simulink model "gm_sampleModel1708_2_sub"  (R2023a)
settings: Solver=VariableStepAuto  StartTime=0.0  StopTime=10.0  RelTol=1e-3
libraries: simulink x4, hdlsllib x1
settings Model: Creator=user1  LastModifiedBy=user1
settings OptimizationCC: BlockReduction=off  ConditionallyExecuteInputs=off
settings DebuggingCC: InheritedTsInSrcMsg=none

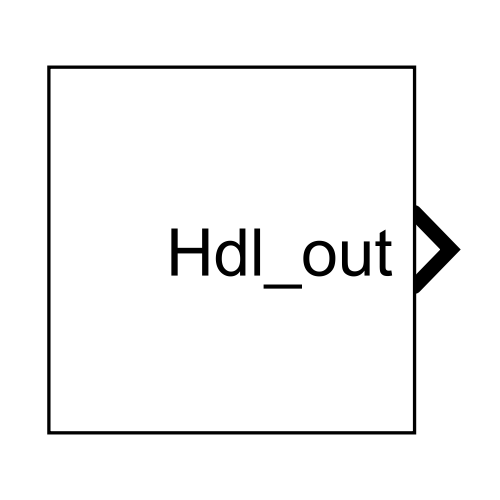
[thumbnail: Simulink's stored preview of the top-level diagram]
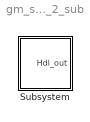
== system gm_sampleModel1708_2_sub ==
  Subsystem : Subsystem

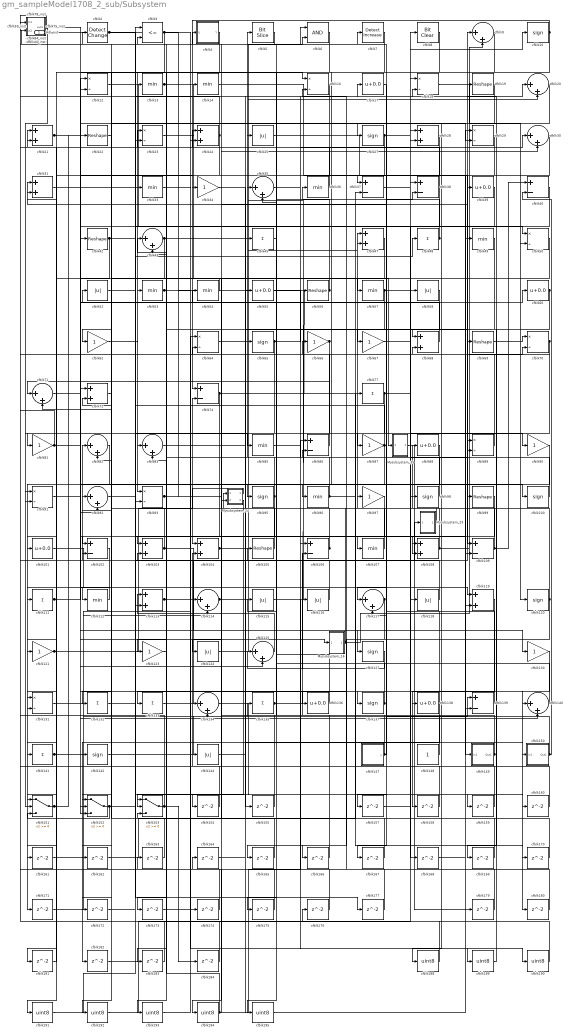
== system gm_sampleModel1708_2_sub/Subsystem ==
  Mysubsystem_16 : Subsystem
  Mysubsystem_23 : Subsystem
  Mysubsystem_24 : Subsystem
  Mysubsystem_35 : Subsystem
  cfblk{10,27,65,95,98,100,120,127,137,142} (10 alike) : Signum
  cfblk{17,39,55,60,88,101,136,138} (8 alike) : Bias  Bias=0.0  SaturateOnIntegerOverflow=off
  cfblk{37..38,40,74,86,102,106,109,139} (9 alike) : Sum  Inputs=+-  OutDataTypeStr=uint8
  cfblk{21,24,28,31,47,68,72,103..104,108,113,119} (12 alike) : Sum  OutDataTypeStr=uint8
  cfblk{19,22,42,56,69,99,105} (7 alike) : Reshape
  cfblk{13..14,33,36,49,53..54,57,85,96,107,112} (12 alike) : MinMax  OutDataTypeStr=uint8
  cfblk{45,48,77,111,132..133,135,141} (8 alike) : Sum  Inputs=+  OutDataTypeStr=uint8
  cfblk{9,20,30,35,43,71,82..83,92,114,117,125,134,140} (14 alike) : Sum  Inputs=|++  OutDataTypeStr=uint8
  cfblk{25,52,58,115..116,118,124,144} (8 alike) : Abs  OutDataTypeStr=uint8  SaturateOnIntegerOverflow=off
  cfblk{12,16,18,23,29,50,64,70,89,91,93,131} (12 alike) : Product  Inputs=*/  OutDataTypeStr=uint8  RndMeth=Zero  SaturateOnIntegerOverflow=on
  cfblk{34,62,66..67,81,87,90,97,121,123,130} (11 alike) : Gain  OutDataTypeStr=uint8
  cfblk122_inst : Subsystem
  cfblk143_inst : Subsystem
  cfblk147 : Subsystem  mask(Counter Limited){uplimit=double(7), tsamp=double(-1)}
      mask prompts: uplimit "Simulink:masks:UpperLimit_MP"; tsamp "Simulink:masks:SampleTime_MP"
      mask help: Simulink:masks:CounterLimited_MD
      mask init:
      | nbits = double(8);
      | tsamp = double(-1);
      | uplimit = double(7);
  cfblk148 : Constant  OutDataTypeStr=uint8  SampleTime=-1
  cfblk149 : Subsystem
  cfblk150 : Subsystem
  cfblk151 : Switch  OutDataTypeStr=uint8  SaturateOnIntegerOverflow=off  InputSameDT=off
  cfblk152 : Switch  OutDataTypeStr=uint8  SaturateOnIntegerOverflow=off  InputSameDT=off
  cfblk153 : Switch  OutDataTypeStr=uint8  SaturateOnIntegerOverflow=off  InputSameDT=off
  cfblk{154..155,157..177,179..184} (29 alike) : Delay  SampleTime=1
  cfblk15_inst : Subsystem
  cfblk{188..195} (8 alike) : DataTypeConversion  OutDataTypeStr=uint8  SaturateOnIntegerOverflow=off  RndMeth=Floor
  cfblk2 : simulink/Logic and Bit Operations/Detect Change  vinit=0  OutDataTypeStr=uint8
      settings: LibrarySourceBlock=|
      | hdlsllib/Logic and Bit
      | Operations/Detect
      | Change
  cfblk26_inst : Subsystem
  cfblk3 : RelationalOperator  Operator=<=  OutDataTypeStr=boolean  InputSameDT=off
  cfblk32_inst : Subsystem
  cfblk4 : Subsystem  mask(Detect Rise Positive){vinit=double(0), InputProcessing=Elements as channels (sample based), OutDataTypeStr=uint8}
      mask prompts: vinit "Simulink:masks:InitialCondition_MP"; InputProcessing "Simulink:masks:InputProcessing_MP"; OutDataTypeStr "Simulink:masks:OutputDataType_MP"
      mask help: Simulink:masks:DetectRisePositive_MD
      mask init:
      | InputProcessing = 'Elements as channels (sample based)';
      | OutDataTypeStr = 'uint8';
      | vinit = double(0);
      mask TypeOptions InputProcessing: Simulink:masks:ColumnsAsChannelsFrameBased | Simulink:masks:ElementsAsChannelsSampleBased
      mask TypeOptions OutDataTypeStr: Simulink:masks:uint8 | Simulink:masks:boolean
      mask Display: fprintf('U > 0\n&  NOT\nU/z > 0')
  cfblk41_inst : Subsystem
  cfblk44_inst : Subsystem
  cfblk5 : hdlsllib/Logic and Bit Operations/Bit Slice  lidx=7  ridx=0
  cfblk51_inst : Subsystem
  cfblk59_inst : Subsystem
  cfblk6 : Logic  AllPortsSameDT=off  OutDataTypeStr=boolean
  cfblk7 : simulink/Logic and Bit Operations/Detect Increase  vinit=0.0  OutDataTypeStr=uint8
      settings: LibrarySourceBlock=|
      | hdlsllib/Logic and Bit
      | Operations/Detect
      | Increase
  cfblk75_inst : Subsystem
  cfblk78_inst : Subsystem
  cfblk8 : simulink/Logic and Bit Operations/Bit Clear  iBit=0
      settings: LibrarySourceBlock=|
      | hdlsllib/Logic and Bit
      | Operations/Bit Clear
  cfblk84_inst : Subsystem
  Hdl_out : Outport  OutDataTypeStr=uint8  SampleTime=1
  wires:
  Mysubsystem_16/1(Out1) -> cfblk9/2, Mysubsystem_24/1(In1)
  Mysubsystem_23/1(Out1) -> cfblk171/1
  Mysubsystem_24/1(Out1) -> cfblk104/1
  Mysubsystem_24/2(Out2) -> cfblk153/2
  Mysubsystem_35/1(Out1) -> cfblk179/1
  cfblk10/1 -> cfblk74/1, cfblk93/1
  cfblk100/1 -> cfblk5/1
  cfblk101/1 -> cfblk119/1
  cfblk102/1 -> cfblk112/1
  cfblk103/1 -> cfblk71/2, cfblk130/1
  cfblk104/1 -> cfblk47/1, cfblk20/2
  cfblk105/1 -> cfblk2/1
  cfblk106/1 -> cfblk43/1, cfblk122_inst/2(in2)
  cfblk107/1 -> cfblk47/2
  cfblk108/1 -> cfblk88/1, cfblk70/2
  cfblk109/1 -> cfblk44_inst/2(in2), cfblk40/1
  cfblk111/1 -> cfblk60/1, Mysubsystem_16/1(In1)
  cfblk112/1 -> cfblk111/1
  cfblk113/1 -> cfblk9/1, Mysubsystem_23/1(In1)
  cfblk114/1 -> cfblk6/2, cfblk77/1
  cfblk115/1 -> cfblk38/2
  cfblk116/1 -> cfblk82/1
  cfblk117/1 -> cfblk166/1, cfblk165/1
  cfblk118/1 -> cfblk51_inst/1(in1)
  cfblk119/1 -> cfblk158/1
  cfblk12/1 -> cfblk168/1
  cfblk120/1 -> cfblk72/2, cfblk133/1
  cfblk121/1 -> cfblk74/2, cfblk181/1
  cfblk122_inst/1(out1) -> cfblk125/2, cfblk57/1
  cfblk123/1 -> cfblk23/1
  cfblk124/1 -> cfblk36/1
  cfblk125/1 -> cfblk113/1
  cfblk127/1 -> cfblk125/1
  cfblk13/1 -> cfblk174/1, cfblk173/1, cfblk45/1
  cfblk130/1 -> cfblk180/1
  cfblk131/1 -> cfblk137/1
  cfblk132/1 -> cfblk159/1
  cfblk133/1 -> cfblk58/1
  cfblk134/1 -> cfblk160/1
  cfblk135/1 -> cfblk56/1, cfblk115/1
  cfblk136/1 -> cfblk35/2
  cfblk137/1 -> cfblk32_inst/1(in1), cfblk31/1
  cfblk138/1 -> cfblk6/1, cfblk41_inst/2(in2), cfblk182/1
  cfblk139/1 -> cfblk35/1
  cfblk14/1 -> cfblk109/1
  cfblk140/1 -> cfblk26_inst/1(in1)
  cfblk141/1 -> cfblk114/2, cfblk23/2
  cfblk142/1 -> cfblk135/1
  cfblk143_inst/1(out1) -> cfblk75_inst/1(in1), cfblk119/2
  cfblk144/1 -> cfblk65/1
  cfblk147/1(y) -> cfblk117/2, cfblk54/1
  cfblk148/1 -> cfblk25/1
  cfblk149/1(Out1) -> cfblk106/2, cfblk66/1
  cfblk15_inst/1(out1) -> cfblk72/1, cfblk50/1
  cfblk150/1(Out1) -> cfblk40/2, cfblk97/1
  cfblk151/1 -> cfblk31/2, cfblk22/1
  cfblk152/1 -> cfblk52/1, cfblk151/3, cfblk105/1
  cfblk153/1 -> cfblk143_inst/2(in2), cfblk184/1
  cfblk154/1 -> cfblk104/2
  cfblk155/1 -> cfblk26_inst/2(in2)
  cfblk157/1 -> cfblk89/2
  cfblk158/1 -> cfblk38/1
  cfblk159/1 -> cfblk86/2
  cfblk16/1 -> cfblk153/1
  cfblk160/1 -> cfblk84_inst/1(in1)
  cfblk161/1 -> cfblk139/1
  cfblk162/1 -> cfblk37/2
  cfblk163/1 -> cfblk153/3
  cfblk164/1 -> cfblk20/1
  cfblk165/1 -> cfblk92/1
  cfblk166/1 -> cfblk3/2
  cfblk167/1 -> cfblk43/2
  cfblk168/1 -> cfblk29/1
  cfblk169/1 -> cfblk24/1
  cfblk17/1 -> cfblk87/1
  cfblk170/1 -> cfblk102/2
  cfblk171/1 -> cfblk64/1
  cfblk172/1 -> cfblk140/2
  cfblk173/1 -> cfblk114/1
  cfblk174/1 -> cfblk75_inst/2(in2)
  cfblk175/1 -> cfblk122_inst/1(in1)
  cfblk176/1 -> cfblk15_inst/2(in2)
  cfblk177/1 -> cfblk103/2
  cfblk179/1 -> cfblk32_inst/2(in2)
  cfblk18/1 -> cfblk120/1
  cfblk180/1 -> cfblk16/2
  cfblk181/1 -> cfblk21/1
  cfblk182/1 -> cfblk28/1
  cfblk183/1 -> cfblk59_inst/1(in1)
  cfblk184/1 -> cfblk78_inst/2(in2)
  cfblk188/1 -> cfblk176/1
  cfblk189/1 -> cfblk19/1
  cfblk19/1 -> cfblk188/1
  cfblk190/1 -> cfblk15_inst/1(in1)
  cfblk191/1 -> cfblk33/1
  cfblk192/1 -> cfblk8/1
  cfblk193/1 -> cfblk134/1
  cfblk194/1 -> cfblk55/1, cfblk116/1, cfblk164/1, cfblk163/1
  cfblk195/1 -> cfblk49/1
  cfblk2/1 -> cfblk177/1, cfblk85/1
  cfblk20/1 -> cfblk102/1
  cfblk21/1 -> cfblk42/1, cfblk50/2
  cfblk22/1 -> cfblk192/1
  cfblk23/1 -> Mysubsystem_35/1(In1)
  cfblk24/1 -> cfblk44_inst/1(in1), cfblk191/1
  cfblk25/1 -> cfblk149/1(In1)
  cfblk26_inst/1(out1) -> cfblk34/1, cfblk29/2
  cfblk27/1 -> cfblk37/1, cfblk10/1
  cfblk28/1 -> cfblk67/1
  cfblk29/1 -> cfblk142/1
  cfblk3/1 -> cfblk24/2, cfblk151/1, cfblk162/1
  cfblk30/1 -> cfblk68/1
  cfblk31/1 -> cfblk18/2
  cfblk32_inst/1(out1) -> cfblk152/2, cfblk140/1
  cfblk33/1 -> cfblk190/1
  cfblk34/1 -> cfblk155/1
  cfblk35/1 -> cfblk17/1
  cfblk36/1 -> cfblk21/2
  cfblk37/1 -> cfblk28/2
  cfblk38/1 -> cfblk59_inst/2(in2), cfblk113/2, cfblk157/1
  cfblk39/1 -> cfblk117/1
  cfblk4/1(Y) -> cfblk123/1
  cfblk40/1 -> cfblk167/1
  cfblk41_inst/1(out1) -> cfblk134/2
  cfblk42/1 -> cfblk108/2, cfblk131/2
  cfblk43/1 -> cfblk69/1, cfblk172/1
  cfblk44_inst/1(out1) -> cfblk12/2
  cfblk45/1 -> cfblk175/1
  cfblk47/1 -> cfblk154/1
  cfblk48/1 -> cfblk18/1, cfblk7/1
  cfblk49/1 -> cfblk194/1
  cfblk5/1 -> cfblk84_inst/2(in2)
  cfblk50/1 -> cfblk103/1
  cfblk51_inst/1(out1) -> cfblk151/2
  cfblk52/1 -> cfblk13/1
  cfblk53/1 -> cfblk144/1, cfblk136/1
  cfblk54/1 -> cfblk53/1
  cfblk55/1 -> cfblk106/1
  cfblk56/1 -> cfblk143_inst/1(in1), Hdl_out/1
  cfblk57/1 -> cfblk83/2, cfblk90/1
  cfblk58/1 -> cfblk107/1
  cfblk59_inst/1(out1) -> cfblk91/1, cfblk16/1
  cfblk6/1 -> cfblk62/1
  cfblk60/1 -> cfblk95/1, cfblk89/1
  cfblk62/1 -> cfblk83/1
  cfblk64/1 -> cfblk150/1(In1)
  cfblk65/1 -> cfblk30/1, cfblk131/1
  cfblk66/1 -> cfblk71/1, cfblk101/1
  cfblk67/1 -> cfblk98/1
  cfblk68/1 -> cfblk12/1
  cfblk69/1 -> cfblk70/1
  cfblk7/1 -> cfblk195/1
  cfblk70/1 -> cfblk68/2, cfblk91/2, cfblk81/1, cfblk169/1
  cfblk71/1 -> cfblk92/2
  cfblk72/1 -> cfblk82/2
  cfblk74/1 -> cfblk138/1, cfblk183/1
  cfblk75_inst/1(out1) -> cfblk99/1, cfblk139/2
  cfblk77/1 -> cfblk152/1, cfblk118/1
  cfblk78_inst/1(out1) -> cfblk100/1
  cfblk8/1 -> cfblk193/1
  cfblk81/1 -> cfblk41_inst/1(in1), cfblk93/2
  cfblk82/1 -> cfblk161/1
  cfblk83/1 -> cfblk108/1
  cfblk84_inst/1(out1) -> cfblk27/1
  cfblk85/1 -> cfblk189/1
  cfblk86/1 -> cfblk64/2
  cfblk87/1 -> cfblk3/1, cfblk109/2, cfblk121/1
  cfblk88/1 -> Mysubsystem_24/2(In2)
  cfblk89/1 -> cfblk78_inst/1(in1)
  cfblk9/1 -> cfblk96/1
  cfblk90/1 -> cfblk141/1
  cfblk91/1 -> cfblk127/1
  cfblk92/1 -> cfblk48/1
  cfblk93/1 -> cfblk39/1, cfblk30/2, cfblk14/1
  cfblk95/1 -> cfblk152/3, cfblk4/1(U)
  cfblk96/1 -> cfblk51_inst/2(in2), cfblk170/1
  cfblk97/1 -> cfblk124/1
  cfblk98/1 -> cfblk86/1
  cfblk99/1 -> cfblk132/1

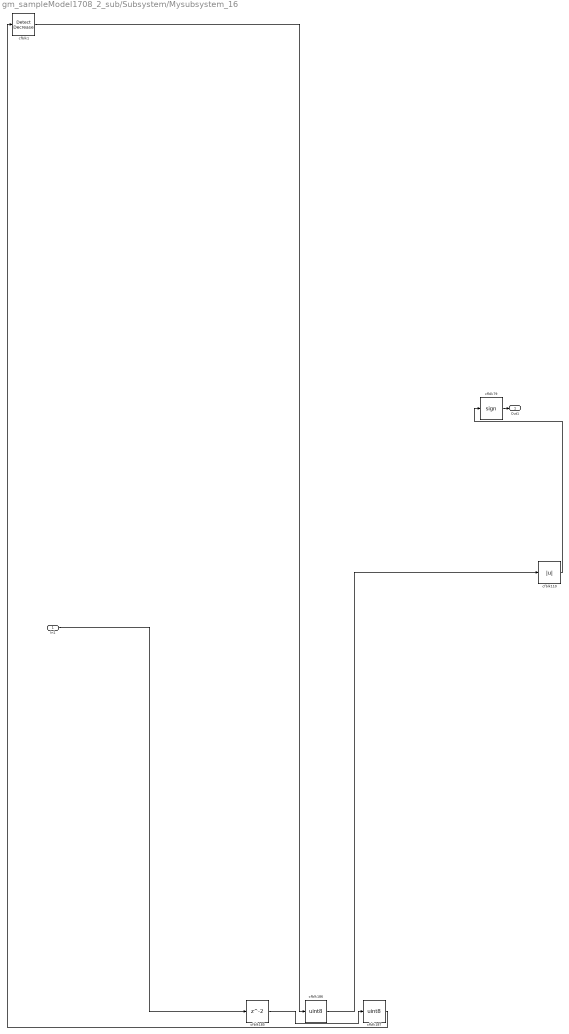
== system gm_sampleModel1708_2_sub/Subsystem/Mysubsystem_16 ==
  In1 : Inport  OutDataTypeStr=uint8  PortDimensions=1  SampleTime=1
  cfblk1 : simulink/Logic and Bit Operations/Detect Decrease  vinit=0.0  OutDataTypeStr=boolean
      settings: LibrarySourceBlock=|
      | hdlsllib/Logic and Bit
      | Operations/Detect
      | Decrease
  cfblk110 : Abs  SaturateOnIntegerOverflow=off
  cfblk185 : Delay  SampleTime=1
  cfblk186 : DataTypeConversion  OutDataTypeStr=uint8  SaturateOnIntegerOverflow=off  RndMeth=Floor
  cfblk187 : DataTypeConversion  OutDataTypeStr=uint8  SaturateOnIntegerOverflow=off  RndMeth=Floor
  cfblk79 : Signum
  Out1 : Outport  SampleTime=1
  wires:
  In1/1 -> cfblk185/1
  cfblk1/1 -> cfblk186/1
  cfblk110/1 -> cfblk79/1
  cfblk185/1 -> cfblk187/1
  cfblk186/1 -> cfblk110/1
  cfblk187/1 -> cfblk1/1
  cfblk79/1 -> Out1/1

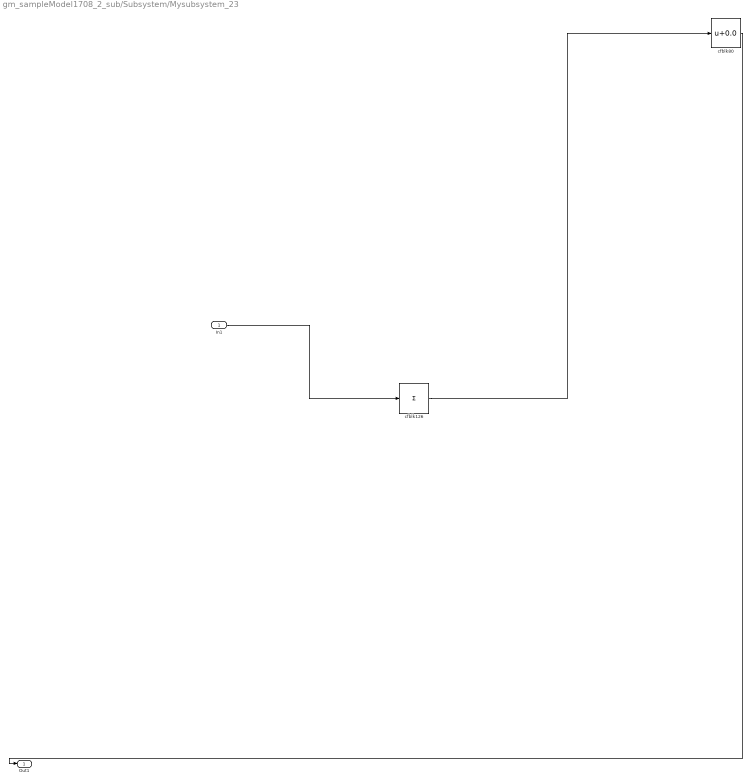
== system gm_sampleModel1708_2_sub/Subsystem/Mysubsystem_23 ==
  In1 : Inport  OutDataTypeStr=uint8  PortDimensions=1  SampleTime=1
  cfblk126 : Sum  Inputs=+
  cfblk80 : Bias  Bias=0.0  SaturateOnIntegerOverflow=off
  Out1 : Outport  SampleTime=1
  wires:
  In1/1 -> cfblk126/1
  cfblk126/1 -> cfblk80/1
  cfblk80/1 -> Out1/1

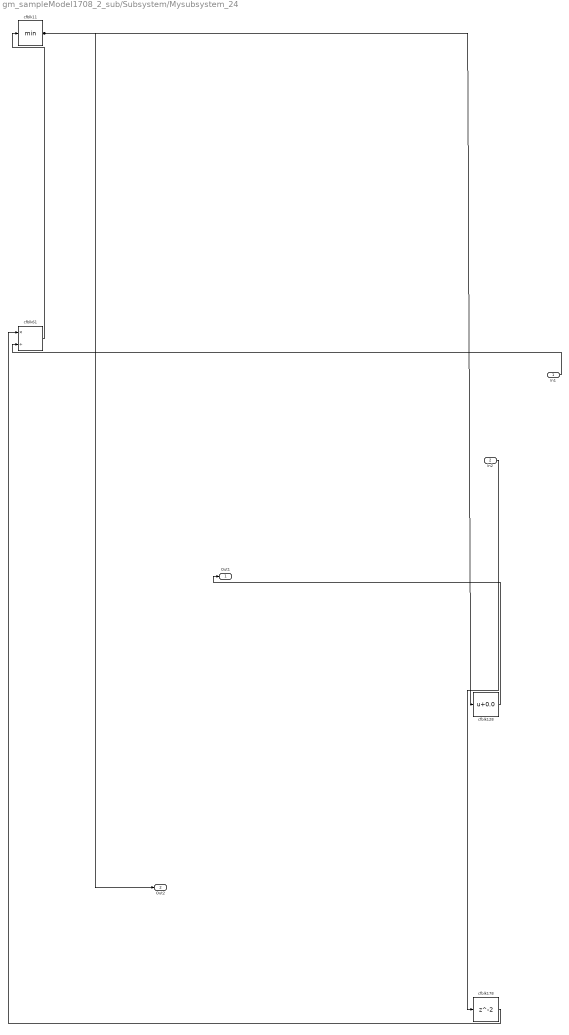
== system gm_sampleModel1708_2_sub/Subsystem/Mysubsystem_24 ==
  In1 : Inport  OutDataTypeStr=uint8  PortDimensions=1  SampleTime=1
  In2 : Inport  Port=2  OutDataTypeStr=uint8  PortDimensions=1  SampleTime=1
  cfblk11 : MinMax
  cfblk128 : Bias  Bias=0.0  SaturateOnIntegerOverflow=off
  cfblk178 : Delay  SampleTime=1
  cfblk61 : Product  Inputs=*/  RndMeth=Zero  SaturateOnIntegerOverflow=on
  Out1 : Outport  SampleTime=1
  Out2 : Outport  Port=2  SampleTime=1
  wires:
  In1/1 -> cfblk61/2
  In2/1 -> cfblk178/1
  cfblk11/1 -> cfblk128/1, Out2/1
  cfblk128/1 -> Out1/1
  cfblk178/1 -> cfblk61/1
  cfblk61/1 -> cfblk11/1

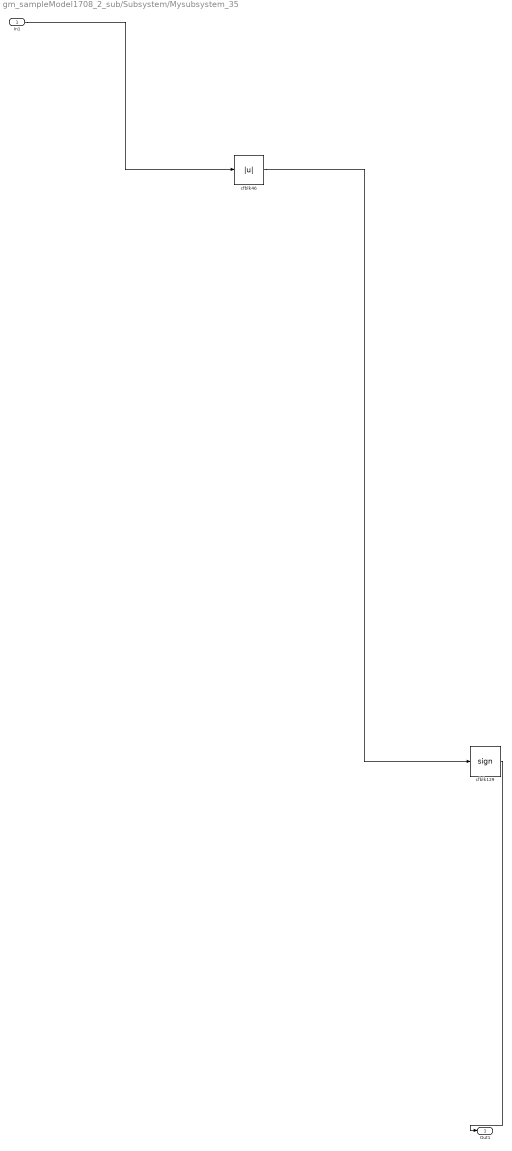
== system gm_sampleModel1708_2_sub/Subsystem/Mysubsystem_35 ==
  In1 : Inport  OutDataTypeStr=uint8  PortDimensions=1  SampleTime=1
  cfblk129 : Signum
  cfblk46 : Abs  SaturateOnIntegerOverflow=off
  Out1 : Outport  SampleTime=1
  wires:
  In1/1 -> cfblk46/1
  cfblk129/1 -> Out1/1
  cfblk46/1 -> cfblk129/1

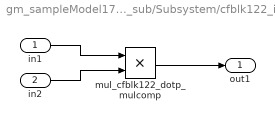
== system gm_sampleModel1708_2_sub/Subsystem/cfblk122_inst ==
  in1 : Inport  OutDataTypeStr=uint8  SampleTime=1
  in2 : Inport  Port=2  OutDataTypeStr=uint8  SampleTime=1
  mul_cfblk122_dotp_mulcomp : Product  Inputs=**  OutDataTypeStr=uint8  SampleTime=1
  out1 : Outport  OutDataTypeStr=uint8  SampleTime=1
  wires:
  in1/1 -> mul_cfblk122_dotp_mulcomp/1
  in2/1 -> mul_cfblk122_dotp_mulcomp/2
  mul_cfblk122_dotp_mulcomp/1 -> out1/1

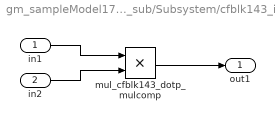
== system gm_sampleModel1708_2_sub/Subsystem/cfblk143_inst ==
  in1 : Inport  OutDataTypeStr=uint8  SampleTime=1
  in2 : Inport  Port=2  OutDataTypeStr=uint8  SampleTime=1
  mul_cfblk143_dotp_mulcomp : Product  Inputs=**  OutDataTypeStr=uint8  SampleTime=1
  out1 : Outport  OutDataTypeStr=uint8  SampleTime=1
  wires:
  in1/1 -> mul_cfblk143_dotp_mulcomp/1
  in2/1 -> mul_cfblk143_dotp_mulcomp/2
  mul_cfblk143_dotp_mulcomp/1 -> out1/1

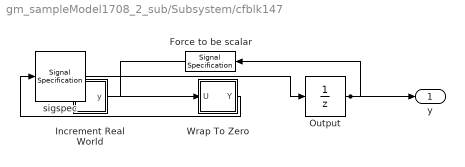
== system gm_sampleModel1708_2_sub/Subsystem/cfblk147 ==
  Force to be scalar : SignalSpecification  DisableCoverage=on  Dimensions=1
  Increment Real World : Subsystem  mask(Real World Value Increment){}
      mask help: Simulink:masks:RealWorldValueIncrement_MD
      mask Display: disp('V++')
  Output : UnitDelay  InitialCondition=0.0  SampleTime=tsamp  HasFrameUpgradeWarning=on
  Wrap To Zero : Subsystem  mask(Wrap To Zero){Threshold=double(7)}
      mask prompts: Threshold "Simulink:masks:Threshold_MP"
      mask help: Simulink:masks:WrapToZero_MD
  sigspec : SignalSpecification  OutDataTypeStr=uint8  Dimensions=1
  y : Outport  SampleTime=1
  wires:
  Force to be scalar/1 -> Increment Real World/1(u)
  Increment Real World/1(y) -> Wrap To Zero/1(U)
  Output/1 -> Force to be scalar/1, y/1
  Wrap To Zero/1(Y) -> sigspec/1
  sigspec/1 -> Output/1

== system gm_sampleModel1708_2_sub/Subsystem/cfblk149 ==
  In1 : Inport  OutDataTypeStr=uint8  PortDimensions=1  SampleTime=1
  Out1 : Outport  SampleTime=1
  wires:
  In1/1 -> Out1/1

== system gm_sampleModel1708_2_sub/Subsystem/cfblk150 ==
  In1 : Inport  OutDataTypeStr=uint8  PortDimensions=1  SampleTime=1
  Out1 : Outport  SampleTime=1
  wires:
  In1/1 -> Out1/1

== system gm_sampleModel1708_2_sub/Subsystem/cfblk15_inst ==
  in1 : Inport  OutDataTypeStr=uint8  SampleTime=1
  in2 : Inport  Port=2  OutDataTypeStr=uint8  SampleTime=1
  mul_cfblk15_dotp_mulcomp : Product  Inputs=**  OutDataTypeStr=uint8  SampleTime=1
  out1 : Outport  OutDataTypeStr=uint8  SampleTime=1
  wires:
  in1/1 -> mul_cfblk15_dotp_mulcomp/1
  in2/1 -> mul_cfblk15_dotp_mulcomp/2
  mul_cfblk15_dotp_mulcomp/1 -> out1/1

== system gm_sampleModel1708_2_sub/Subsystem/cfblk26_inst ==
  in1 : Inport  OutDataTypeStr=uint8  SampleTime=1
  in2 : Inport  Port=2  OutDataTypeStr=uint8  SampleTime=1
  mul_cfblk26_dotp_mulcomp : Product  Inputs=**  OutDataTypeStr=uint8  SampleTime=1
  out1 : Outport  OutDataTypeStr=uint8  SampleTime=1
  wires:
  in1/1 -> mul_cfblk26_dotp_mulcomp/1
  in2/1 -> mul_cfblk26_dotp_mulcomp/2
  mul_cfblk26_dotp_mulcomp/1 -> out1/1

== system gm_sampleModel1708_2_sub/Subsystem/cfblk32_inst ==
  in1 : Inport  OutDataTypeStr=uint8  SampleTime=1
  in2 : Inport  Port=2  OutDataTypeStr=uint8  SampleTime=1
  mul_cfblk32_dotp_mulcomp : Product  Inputs=**  OutDataTypeStr=uint8  SampleTime=1
  out1 : Outport  OutDataTypeStr=uint8  SampleTime=1
  wires:
  in1/1 -> mul_cfblk32_dotp_mulcomp/1
  in2/1 -> mul_cfblk32_dotp_mulcomp/2
  mul_cfblk32_dotp_mulcomp/1 -> out1/1

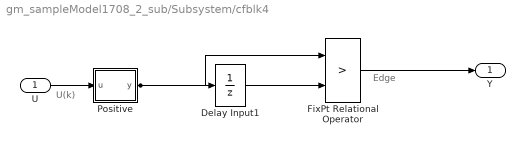
== system gm_sampleModel1708_2_sub/Subsystem/cfblk4 ==
  note: U(k)
  note: Edge
  U : Inport  OutDataTypeStr=uint8  SampleTime=1
  Delay Input1 : UnitDelay  Description=Store in Global RAM  DisableCoverage=on  InitialCondition=vinit  SampleTime=-1  HasFrameUpgradeWarning=on
  FixPt Relational Operator : RelationalOperator  Operator=>  OutDataTypeStr=fixdt(0, 8)  ZeroCross=off  InputSameDT=off
  Positive : Subsystem  mask(Compare To Zero){relop=>, OutDataTypeStr=boolean, ZeroCross=off}
      mask prompts: relop "Simulink:masks:Operator_MP"; OutDataTypeStr "Simulink:masks:OutputDataType_MP"; ZeroCross "Simulink:masks:EnableZerocrossingDetection_MP"
      mask help: Simulink:masks:CompareToZero_MD
      mask init:
      | OutDataTypeStr = 'boolean';
      | ZeroCross = 'off';
      | blkName = 'sampleModel1708_2_sub/Subsystem/cfblk4/Positive';
      | relop = '>';
      | setValue = 'boolean';
      mask TypeOptions relop: == | ~= | < | <= | >= | >
      mask TypeOptions OutDataTypeStr: Simulink:masks:uint8 | Simulink:masks:boolean
      mask Callback ZeroCross: sl('zeroCrossEnable', gcbh);
      mask Display: disp([relop,' 0'])
  Y : Outport  SampleTime=1
  wires:
  U/1 -> Positive/1(u)
  Delay Input1/1 -> FixPt Relational Operator/2
  FixPt Relational Operator/1 -> Y/1
  Positive/1(y) -> FixPt Relational Operator/1, Delay Input1/1

== system gm_sampleModel1708_2_sub/Subsystem/cfblk41_inst ==
  in1 : Inport  OutDataTypeStr=uint8  SampleTime=1
  in2 : Inport  Port=2  OutDataTypeStr=uint8  SampleTime=1
  mul_cfblk41_dotp_mulcomp : Product  Inputs=**  OutDataTypeStr=uint8  SampleTime=1
  out1 : Outport  OutDataTypeStr=uint8  SampleTime=1
  wires:
  in1/1 -> mul_cfblk41_dotp_mulcomp/1
  in2/1 -> mul_cfblk41_dotp_mulcomp/2
  mul_cfblk41_dotp_mulcomp/1 -> out1/1

== system gm_sampleModel1708_2_sub/Subsystem/cfblk44_inst ==
  in1 : Inport  OutDataTypeStr=uint8  SampleTime=1
  in2 : Inport  Port=2  OutDataTypeStr=uint8  SampleTime=1
  mul_cfblk44_dotp_mulcomp : Product  Inputs=**  OutDataTypeStr=uint8  SampleTime=1
  out1 : Outport  OutDataTypeStr=uint8  SampleTime=1
  wires:
  in1/1 -> mul_cfblk44_dotp_mulcomp/1
  in2/1 -> mul_cfblk44_dotp_mulcomp/2
  mul_cfblk44_dotp_mulcomp/1 -> out1/1

== system gm_sampleModel1708_2_sub/Subsystem/cfblk51_inst ==
  in1 : Inport  OutDataTypeStr=uint8  SampleTime=1
  in2 : Inport  Port=2  OutDataTypeStr=uint8  SampleTime=1
  mul_cfblk51_dotp_mulcomp : Product  Inputs=**  OutDataTypeStr=uint8  SampleTime=1
  out1 : Outport  OutDataTypeStr=uint8  SampleTime=1
  wires:
  in1/1 -> mul_cfblk51_dotp_mulcomp/1
  in2/1 -> mul_cfblk51_dotp_mulcomp/2
  mul_cfblk51_dotp_mulcomp/1 -> out1/1

== system gm_sampleModel1708_2_sub/Subsystem/cfblk59_inst ==
  in1 : Inport  OutDataTypeStr=uint8  SampleTime=1
  in2 : Inport  Port=2  OutDataTypeStr=uint8  SampleTime=1
  mul_cfblk59_dotp_mulcomp : Product  Inputs=**  OutDataTypeStr=uint8  SampleTime=1
  out1 : Outport  OutDataTypeStr=uint8  SampleTime=1
  wires:
  in1/1 -> mul_cfblk59_dotp_mulcomp/1
  in2/1 -> mul_cfblk59_dotp_mulcomp/2
  mul_cfblk59_dotp_mulcomp/1 -> out1/1

== system gm_sampleModel1708_2_sub/Subsystem/cfblk75_inst ==
  in1 : Inport  OutDataTypeStr=uint8  SampleTime=1
  in2 : Inport  Port=2  OutDataTypeStr=uint8  SampleTime=1
  mul_cfblk75_dotp_mulcomp : Product  Inputs=**  OutDataTypeStr=uint8  SampleTime=1
  out1 : Outport  OutDataTypeStr=uint8  SampleTime=1
  wires:
  in1/1 -> mul_cfblk75_dotp_mulcomp/1
  in2/1 -> mul_cfblk75_dotp_mulcomp/2
  mul_cfblk75_dotp_mulcomp/1 -> out1/1

== system gm_sampleModel1708_2_sub/Subsystem/cfblk78_inst ==
  in1 : Inport  OutDataTypeStr=uint8  SampleTime=1
  in2 : Inport  Port=2  OutDataTypeStr=uint8  SampleTime=1
  mul_cfblk78_dotp_mulcomp : Product  Inputs=**  OutDataTypeStr=uint8  SampleTime=1
  out1 : Outport  OutDataTypeStr=uint8  SampleTime=1
  wires:
  in1/1 -> mul_cfblk78_dotp_mulcomp/1
  in2/1 -> mul_cfblk78_dotp_mulcomp/2
  mul_cfblk78_dotp_mulcomp/1 -> out1/1

== system gm_sampleModel1708_2_sub/Subsystem/cfblk84_inst ==
  in1 : Inport  OutDataTypeStr=uint8  SampleTime=1
  in2 : Inport  Port=2  OutDataTypeStr=uint8  SampleTime=1
  mul_cfblk84_dotp_mulcomp : Product  Inputs=**  OutDataTypeStr=uint8  SampleTime=1
  out1 : Outport  OutDataTypeStr=uint8  SampleTime=1
  wires:
  in1/1 -> mul_cfblk84_dotp_mulcomp/1
  in2/1 -> mul_cfblk84_dotp_mulcomp/2
  mul_cfblk84_dotp_mulcomp/1 -> out1/1

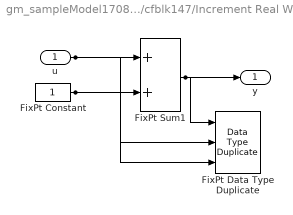
== system gm_sampleModel1708_2_sub/Subsystem/cfblk147/Increment Real World ==
  u : Inport  OutDataTypeStr=uint8  SampleTime=1
  FixPt Constant : Constant  DisableCoverage=on  OutDataTypeStr=Inherit: Inherit via back propagation  SampleTime=-1
  FixPt Data Type Duplicate : DataTypeDuplicate  DisableCoverage=on  NumInputPorts=3
  FixPt Sum1 : Sum  InputSameDT=on  OutDataTypeStr=Inherit: Inherit via back propagation  LockScale=on
  y : Outport  SampleTime=1
  wires:
  u/1 -> FixPt Sum1/1, FixPt Data Type Duplicate/2
  FixPt Constant/1 -> FixPt Sum1/2, FixPt Data Type Duplicate/3
  FixPt Sum1/1 -> FixPt Data Type Duplicate/1, y/1

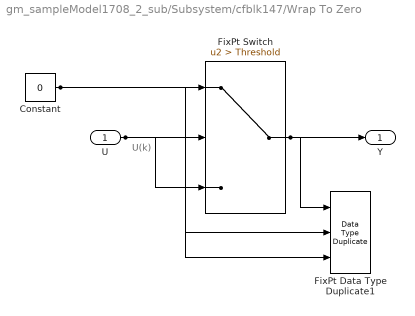
== system gm_sampleModel1708_2_sub/Subsystem/cfblk147/Wrap To Zero ==
  note: U(k)
  U : Inport  OutDataTypeStr=uint8  SampleTime=1
  Constant : Constant  DisableCoverage=on  Value=0  OutDataTypeStr=Inherit: Inherit via back propagation  SampleTime=-1
  FixPt Data Type Duplicate1 : DataTypeDuplicate  DisableCoverage=on  NumInputPorts=3
  FixPt Switch : Switch  Criteria=u2 > Threshold  Threshold=Threshold  OutDataTypeStr=Inherit: Inherit via back propagation  ZeroCross=off  SaturateOnIntegerOverflow=off  InputSameDT=off
  Y : Outport  SampleTime=1
  wires:
  U/1 -> FixPt Switch/3, FixPt Switch/2, FixPt Data Type Duplicate1/2
  Constant/1 -> FixPt Switch/1, FixPt Data Type Duplicate1/3
  FixPt Switch/1 -> FixPt Data Type Duplicate1/1, Y/1

== system gm_sampleModel1708_2_sub/Subsystem/cfblk4/Positive ==
  u : Inport  OutDataTypeStr=uint8  SampleTime=1
  Compare : RelationalOperator  Operator=>  OutDataTypeStr=boolean  ZeroCross=off
  Constant : Constant  DisableCoverage=on  Value=0  OutDataTypeStr=Inherit: Inherit via back propagation  SampleTime=-1  PreserveConstantTs=on
  y : Outport  SampleTime=1
  wires:
  u/1 -> Compare/1
  Compare/1 -> y/1
  Constant/1 -> Compare/2
